simulink model "TP4_2015b"  (R2015b)
settings: Solver=VariableStepAuto  SolverMode=SingleTasking  StartTime=0.0  StopTime=30  RelTol=1e-3
values from neighbouring files (symbols this model uses):
  Alat = [Ybeta/u0 Yp/u0 -(1-Yr/u0) (g/u0)*cos(theta0) ... (first row only)    [labo4clement.m]
  Alon = [Xu              Xw              0               -g*cos(theta0) ... (first row only)    [labo4clement.m]
  Blat = [Ygamaileron/u0 Ygamrudder/u0 ... (first row only)    [labo4clement.m]
  Blon = [Xgamaelevator ... (first row only)    [labo4clement.m]
  Clat = eye(4,4)    [labo4clement.m]
  Clon = eye(4,4)    [labo4clement.m]
  Dlat = [0 0; 0 0; 0 0; 0 0]    [labo4clement.m]
  Dlon = [0; 0; 0; 0]    [labo4clement.m]
undefined symbols (not defined in the file or in its folder): sigbuilder_block
libraries: simulink x1
settings Model: Creator=AP19030  LastModifiedBy=AP19030
settings DataIOCC: LimitDataPoints=off
settings DebuggingCC: AllowSymbolicDim=on  SFUnexpectedBacktrackingDiag=error  SFNoUnconditionalDefaultTransitionDiag=error
settings ModelReferenceCC: PropagateSignalLabelsOutOfModel=on
settings GRTTargetCC: TargetLangStandard=C99 (ISO)
settings ConfigComp: CovMetricSettings=dwe  CovHtmlReporting=off  CovSaveCumulativeToWorkspaceVar=off  CovSaveSingleToWorkspaceVar=off  CovModelRefEnable=Off  CovExternalEMLEnable=on

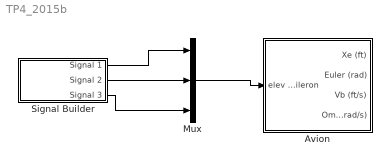
== system TP4_2015b ==
  Avion : Subsystem
  Mux : Mux  Inputs=3
  Signal Builder : Subsystem  Tag=STV Subsys  LoadFcn=sigbuilder_block('load');  StartFcn=sigbuilder_block('start');  StopFcn=sigbuilder_block('stop');  ClipboardFcn=sigbuilder_block('clipboard');  mask(Sigbuilder block){}
      mask help: Simulink:masks:SigbuilderBlock_MD
      mask init:
      | if ~strcmp(get_param(bdroot(gcbh),'SimulationStatus'),'stopped') tuvar = sigbuilder_block('maskInit'); end
      settings: CopyFcn=sigbuilder_block('copy');  DeleteFcn=sigbuilder_block('delete');  ModelCloseFcn=sigbuilder_block('modelClose');  PreSaveFcn=sigbuilder_block('preSave');  PauseFcn=sigbuilder_block('pause');  ContinueFcn=sigbuilder_block('continue');  NameChangeFcn=sigbuilder_block('namechange');  OpenFcn=sigbuilder_block('open',[60.75 183 550.5 399.75 ]);  CloseFcn=sigbuilder_block('close');
      mask Display: plot(0, 0, 100, 100,[2, 2, 32, 32, 2], [68, 8, 8, 68, 68],[32, 2], [38, 38], [32, 19, 2],[53, 60, 44], [32, 17, 17, 2],[16, 16, 31, 31]);txt = getActiveGroup(gcbh);text(2, 100, txt,'verticalAlignment', 'top');
  wires:
  Signal Builder/2(Signal 2) -> Mux/2
  Signal Builder/1(Signal 1) -> Mux/1
  Signal Builder/3(Signal 3) -> Mux/3
  Mux/1 -> Avion/1(elev aileron)

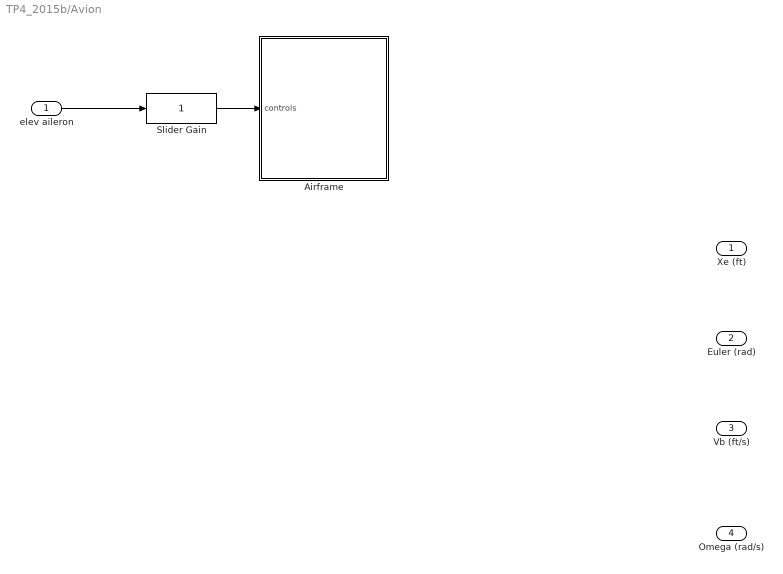
== system TP4_2015b/Avion ==
  elev aileron : Inport
  Airframe : Subsystem
  Slider Gain : simulink/Math Operations/Slider Gain  low=0  gain=1  high=2
  Xe (ft) : Outport
  Euler (rad) : Outport  Port=2
  Vb (ft/s) : Outport  Port=3
  Omega (rad/s) : Outport  Port=4
  wires:
  elev aileron/1 -> Slider Gain/1
  ? -> ?
  ? -> Xe (ft)/1
  ? -> Euler (rad)/1
  ? -> Vb (ft/s)/1
  ? -> Omega (rad/s)/1
  Slider Gain/1 -> Airframe/1(controls)

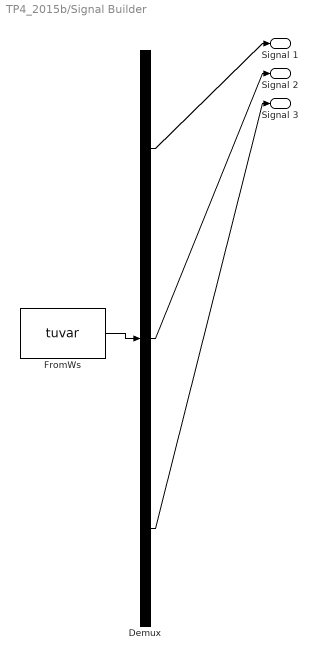
== system TP4_2015b/Signal Builder ==
  Demux : Demux  Tag=STV Demux  Outputs=3
  FromWs : FromWorkspace  Tag=STV FromWs  VariableName=tuvar  SampleTime=0
      SigBuilderData=|
      | common.afterFinalStr = 'Extrapolate'
      | common.sampleTime = 0
      | dataSet.timeRange = [0 30]
      | dataSet.name = 'Group 1'
      | sbobj.Groups.Name = 'Group 1'
      | sbobj.Groups.Signals(1).Name = 'Signal 1'
      | sbobj.Groups.Signals(1).XData = [0 1 1 1.1 1.1 5 5 5.1 5.1 30]
      | sbobj.Groups.Signals(1).YData = [0 0 1 1 0 0 -1 -1 0 0]
      | sbobj.Groups.Signals(2).Name = 'Signal 2'
      | sbobj.Groups.Signals(2).XData = [0 10.1 10.1 10.2 10.2 15.05 15.05 15.15 15.15 30]
      | sbobj.Groups.Signals(2).YData = [0 0 1 1 0 0 -1 -1 0 0]
      | sbobj.Groups.Signals(3).Name = 'Signal 3'
      | sbobj.Groups.Signals(3).XData = [0 19.95 19.95 20.1 20.1 25 25 25.1 25.1 30]
      | sbobj.Groups.Signals(3).YData = [0 0 1 1 0 0 -1 -1 0 0]
      | sbobj.Groups.TimeRange = [0 30]
  Signal 1 : Outport  Tag=STV Outport
  Signal 2 : Outport  Tag=STV Outport  Port=2
  Signal 3 : Outport  Tag=STV Outport  Port=3
  wires:
  FromWs/1 -> Demux/1
  Demux/1 -> Signal 1/1
  Demux/2 -> Signal 2/1
  Demux/3 -> Signal 3/1

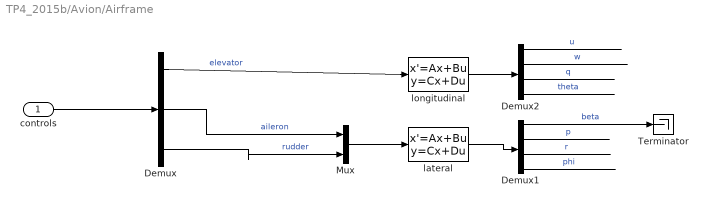
== system TP4_2015b/Avion/Airframe ==
  controls : Inport
  Demux : Demux  Outputs=3
  Demux1 : Demux
  Demux2 : Demux
  Mux : Mux  Inputs=2
  Terminator : Terminator
  lateral : StateSpace  A=Alat  B=Blat  C=Clat  D=Dlat  X0=0
  longitudinal : StateSpace  A=Alon  B=Blon  C=Clon  D=Dlon  X0=0
  wires:
  controls/1 -> Demux/1
  Demux/1 -> longitudinal/1  "elevator"
  Demux/2 -> Mux/1  "aileron"
  Demux/3 -> Mux/2  "rudder"
  Mux/1 -> lateral/1
  lateral/1 -> Demux1/1
  longitudinal/1 -> Demux2/1
  Demux2/1 -> ?  "u"
  Demux2/2 -> ?  "w"
  Demux2/3 -> ?  "q"
  Demux2/4 -> ?  "theta"
  Demux1/1 -> Terminator/1  "beta"
  Demux1/2 -> ?  "p"
  Demux1/3 -> ?  "r"
  Demux1/4 -> ?  "phi"
